simulink model "SingleVehicle_01"  (Simulink 8.8)
settings: Solver=ode45  StartTime=0.0  StopTime=17  RelTol=1e-3  EnableMultiTasking=on
undefined symbols (not defined in the file or in its folder): DiscIntNeverNeededParam, dpsi, FromPrescan, IdealSensors, psi, RHSC, RHSCCmdBus, unscented_KF_dd, v, wpFollower, y
undefined symbols (not defined in the file): vd
libraries: commchan3 x4
settings Model: Creator=sgopalswamy  LastModifiedBy=yutongli
settings SolverCC: AutoInsertRateTranBlk=on
settings DataIOCC: LimitDataPoints=off  SaveFormat=Dataset  SignalLoggingSaveFormat=Dataset
settings OptimizationCC: LifeSpan=auto
settings DebuggingCC: MultiTaskRateTransMsg=warning  FcnCallInpInsideContextMsg=error  StateNameClashWarn=none  SFUnexpectedBacktrackingDiag=error  SFNoUnconditionalDefaultTransitionDiag=error
settings HardwareCC: ProdBitPerPointer=64  ProdBitPerSizeT=64  ProdBitPerPtrDiffT=64  ProdLargestAtomicFloat=Float  ProdIntDivRoundTo=Zero  ProdEndianess=LittleEndian  ProdWordSize=64  ProdHWDeviceType=Intel->x86-64 (Windows64)
settings ModelReferenceCC: PropagateSignalLabelsOutOfModel=on
settings GRTTargetCC: TargetLangStandard=C99 (ISO)  GeneratePreprocessorConditionals=Use local settings  CombineOutputUpdateFcns=on  GRTInterface=off
settings ConfigComp: CovSFcnEnable=off

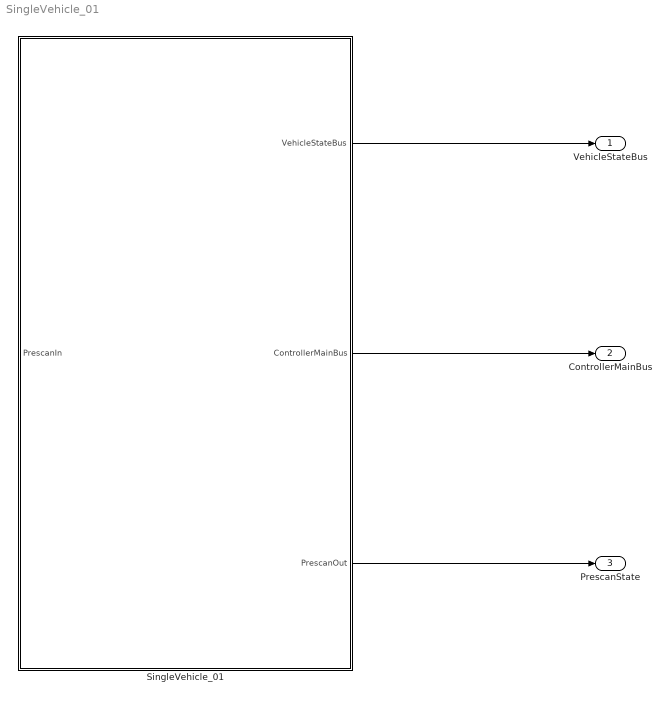
== system SingleVehicle_01 ==
  SingleVehicle_01 : Subsystem  mask{veh_struct=vd}
      mask prompts: veh_struct "Vehicle Parameter Structure"
      mask init:
      | set_param([gcb,'/Monitor/VehicleStateBusStorage'],'VariableName',[get_param(gcb,'MaskValueString'),'_DataVehicleBus']);
      | set_param([gcb,'/Monitor/ControllerMainBusStorage/ArbitratedActuationReqStorage'],'VariableName', ...
      |     [get_param(gcb,'MaskValueString'),'_DataControllerMain_ArbitrationActuationReq']);
      | set_param([gcb,'/Monitor/ControllerMainBusStorage/wpFollowerStorage'],'VariableName', ...
      |     [get_param(gcb,'MaskValueString'),'_DataControllerMain_wpFollower']);
      | set_param([gcb,'/Monitor/ControllerMainBusStorage/finalWayPointStorarge'],'VariableName', ...
      |     [get_param(gcb,'MaskValueString'),'_DataControllerMain_finalWayPoint']);
      | set_param([gcb,'/Monitor/ControllerMainBusStorage/currentWayPointStorage'],'VariableName', ...
      |     [get_param(gcb,'MaskValueString'),'_DataControllerMain_currentWayPoint']);
      | set_param([gcb,'/Monitor/ControllerMainBusStorage/wayPointArrayStorage'],'VariableName', ...
      |     [get_param(gcb,'MaskValueString'),'_DataControllerMain_wayPointArray']);
      | set_param([gcb,'/Monitor/ControllerMainBusStorage/selfAwareessBusStorage'],'VariableName', ...
      |     [get_param(gcb,'MaskValueString'),'_DataControllerMain_selfAwareessBus']);
      | set_param([gcb,'/Monitor/ControllerMainBusStorage/IdealSensorsStorage'],'VariableName', ...
      |     [get_param(gcb,'MaskValueString'),'_DataControllerMain_IdealSensors']);
      | set_param([gcb,'/Monitor/ControllerMainBusStorage/FromPrescanStorage'],'VariableName', ...
      |     [get_param(gcb,'MaskValueString'),'_DataControllerMain_FromPrescan']);
  VehicleStateBus : Outport
  ControllerMainBus : Outport  Port=2
  PrescanState : Outport  Port=3
  wires:
  SingleVehicle_01/1(VehicleStateBus) -> VehicleStateBus/1
  SingleVehicle_01/2(ControllerMainBus) -> ControllerMainBus/1
  SingleVehicle_01/3(PrescanOut) -> PrescanState/1

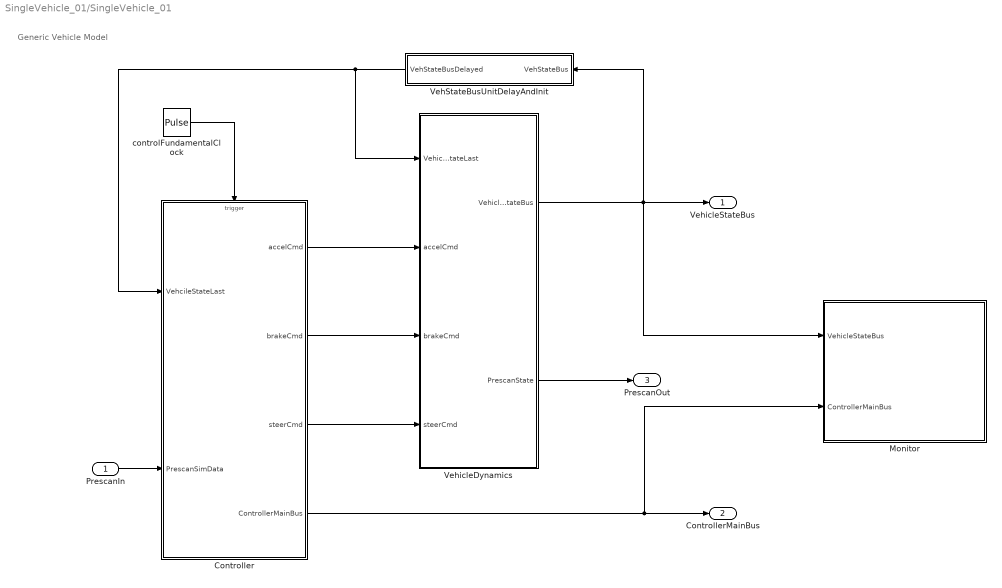
== system SingleVehicle_01/SingleVehicle_01 ==
  note: Generic Vehicle Model
  PrescanIn : Inport
  Controller : Subsystem
  Monitor : Subsystem
  VehStateBusUnitDelayAndInit : Subsystem
  VehicleDynamics : Subsystem
  controlFundamentalClock : DiscretePulseGenerator  PulseType=Time based  Period=veh_struct.CONTROL_OS_SAMPLETIME  PulseWidth=5
  VehicleStateBus : Outport
  ControllerMainBus : Outport  Port=2
  PrescanOut : Outport  Port=3
  wires:
  PrescanIn/1 -> Controller/2(PrescanSimData)
  Controller/1(accelCmd) -> VehicleDynamics/2(accelCmd)
  Controller/2(brakeCmd) -> VehicleDynamics/3(brakeCmd)
  Controller/3(steerCmd) -> VehicleDynamics/4(steerCmd)
  Controller/4(ControllerMainBus) -> Monitor/2(ControllerMainBus), ControllerMainBus/1
  VehicleDynamics/2(PrescanState) -> PrescanOut/1
  VehicleDynamics/1(VehicleStateBus) -> Monitor/1(VehicleStateBus), VehicleStateBus/1, VehStateBusUnitDelayAndInit/1(VehStateBus)
  VehStateBusUnitDelayAndInit/1(VehStateBusDelayed) -> VehicleDynamics/1(VehicleStateLast), Controller/1(VehcileStateLast)
  controlFundamentalClock/1 -> Controller/Trigger

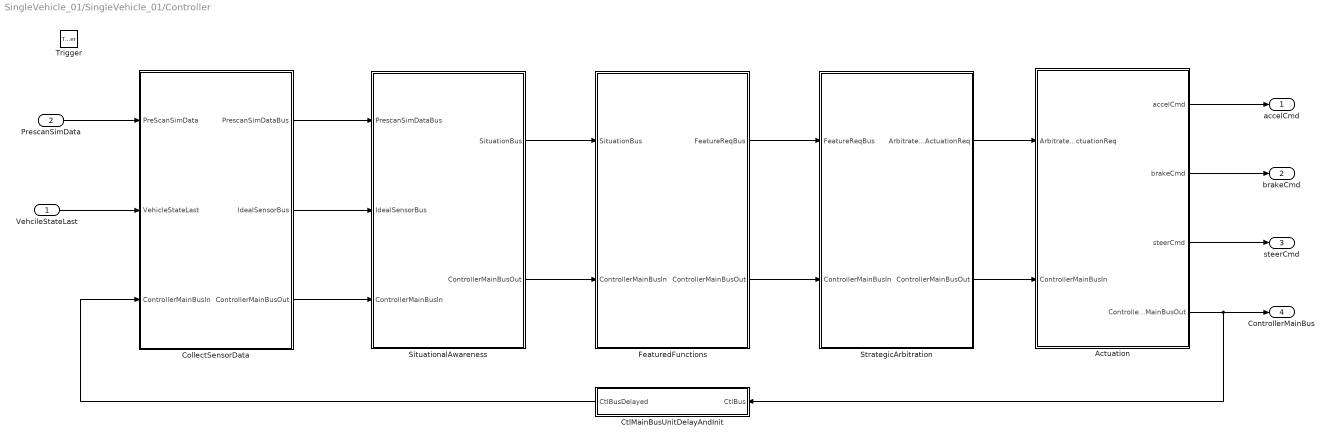
== system SingleVehicle_01/SingleVehicle_01/Controller ==
  VehcileStateLast : Inport
  PrescanSimData : Inport  Port=2
  Trigger : TriggerPort  VariantControl=Variant  PortDimensions=1
  Actuation : Subsystem
  CollectSensorData : Subsystem
  CtlMainBusUnitDelayAndInit : Subsystem
  FeaturedFunctions : Subsystem
  SituationalAwareness : Subsystem
  StrategicArbitration : Subsystem
  accelCmd : Outport
  brakeCmd : Outport  Port=2
  steerCmd : Outport  Port=3
  ControllerMainBus : Outport  Port=4
  wires:
  PrescanSimData/1 -> CollectSensorData/1(PreScanSimData)
  Actuation/1(accelCmd) -> accelCmd/1
  Actuation/2(brakeCmd) -> brakeCmd/1
  Actuation/3(steerCmd) -> steerCmd/1
  StrategicArbitration/1(ArbitratedActuationReq) -> Actuation/1(ArbitratedActuationReq)
  StrategicArbitration/2(ControllerMainBusOut) -> Actuation/2(ControllerMainBusIn)
  FeaturedFunctions/2(ControllerMainBusOut) -> StrategicArbitration/2(ControllerMainBusIn)
  FeaturedFunctions/1(FeatureReqBus) -> StrategicArbitration/1(FeatureReqBus)
  SituationalAwareness/1(SituationBus) -> FeaturedFunctions/1(SituationBus)
  SituationalAwareness/2(ControllerMainBusOut) -> FeaturedFunctions/2(ControllerMainBusIn)
  CollectSensorData/3(ControllerMainBusOut) -> SituationalAwareness/3(ControllerMainBusIn)
  VehcileStateLast/1 -> CollectSensorData/2(VehicleStateLast)
  Actuation/4(ControllerMainBusOut) -> CtlMainBusUnitDelayAndInit/1(CtlBus), ControllerMainBus/1
  CtlMainBusUnitDelayAndInit/1(CtlBusDelayed) -> CollectSensorData/3(ControllerMainBusIn)
  CollectSensorData/1(PrescanSimDataBus) -> SituationalAwareness/1(PrescanSimDataBus)
  CollectSensorData/2(IdealSensorBus) -> SituationalAwareness/2(IdealSensorBus)

== system SingleVehicle_01/SingleVehicle_01/Monitor ==
  VehicleStateBus : Inport
  ControllerMainBus : Inport  Port=2
  ControllerMainBusStorage : Subsystem
  VehicleStateBusStorage : ToWorkspace  VariableName=vd_DataVehicleBus  SaveFormat=Timeseries  SampleTime=-1
  wires:
  VehicleStateBus/1 -> VehicleStateBusStorage/1
  ControllerMainBus/1 -> ControllerMainBusStorage/1(ControllerMainBus)

== system SingleVehicle_01/SingleVehicle_01/VehStateBusUnitDelayAndInit ==
  VehStateBus : Inport
  MATLAB Function : MATLAB Function  TreatAsAtomicUnit=on
  Memory : Memory  InheritSampleTime=on
  VehStateBusDelayed : Outport
  wires:
  Memory/1 -> MATLAB Function/1(u)
  VehStateBus/1 -> Memory/1
  MATLAB Function/1(y) -> VehStateBusDelayed/1

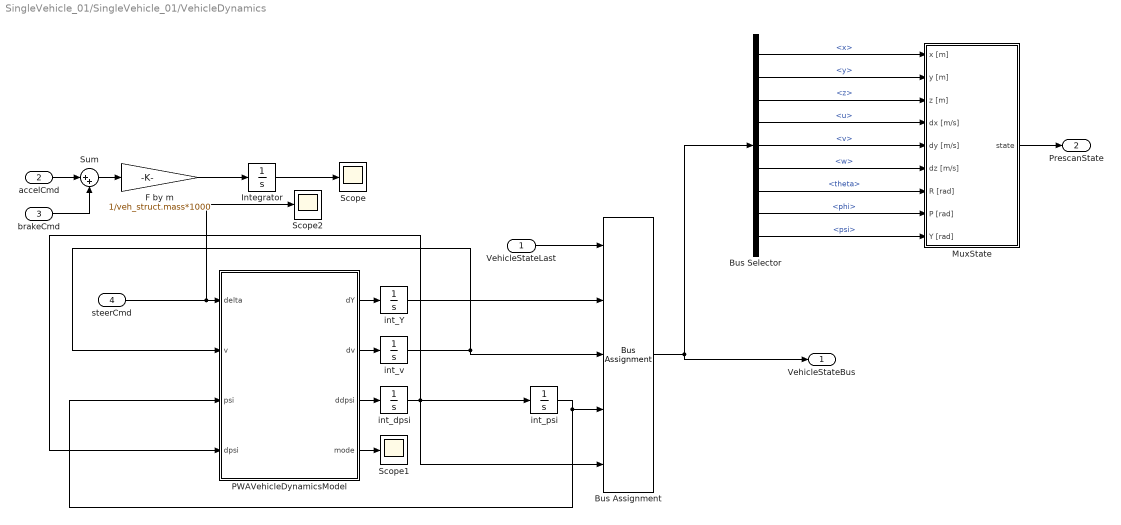
== system SingleVehicle_01/SingleVehicle_01/VehicleDynamics ==
  VehicleStateLast : Inport
  accelCmd : Inport  Port=2
  brakeCmd : Inport  Port=3
  steerCmd : Inport  Port=4
  Bus Assignment : BusAssignment  AssignedSignals=y,v,psi,dpsi
  Bus Selector : BusSelector  OutputSignals=x,y,z,u,v,w,theta,phi,psi
  F by m : Gain  Gain=1/veh_struct.mass*1000
  Integrator : Integrator  InitialCondition=veh_struct.init.u
  MuxState : Subsystem  Tag=MuxState  mask(Empty Dynamics State Block){positioningmode=on, TimeStep=1/20}
      mask prompts: positioningmode "Positioning Mode"; TimeStep "Auto Assigned: Time Step [s]"
      mask help:
      | Build the state of an actor based on user input.
      | The user can either use positioning mode or dynamics mode.
      | - When using positioning mode the position and orientation of the actor are set directly based on the input. Expected input is relative to the initial position and orientation of the actor. It's also possible to specify the velocity of the actor, though this input isn't used, only passed on.
      | - When using dynamics mode the position input is ignored. Expected input is velocity and orientation. The velocity is relative the current orientation of the actor, while orientation is relative to its initial orientation. The position of the actor is calculated based on the velocity and orientation given.
      settings: DeleteFcn=PreScanBlockDeleteFcn;
  PWAVehicleDynamicsModel : MATLAB Function  TreatAsAtomicUnit=on
  Scope : Scope
  Scope1 : Scope
  Scope2 : Scope
  Sum : Sum  Inputs=|++
  int_Y : Integrator  InitialCondition=veh_struct.init.Y
  int_dpsi : Integrator  InitialCondition=veh_struct.init.dpsi
  int_psi : Integrator  InitialCondition=veh_struct.init.psi
  int_v : Integrator  InitialCondition=veh_struct.init.v
  VehicleStateBus : Outport
  PrescanState : Outport  Port=2
  wires:
  MuxState/1(state) -> PrescanState/1
  Bus Assignment/1 -> VehicleStateBus/1, Bus Selector/1
  Bus Selector/3 -> MuxState/3(z [m])  "<z>"
  Bus Selector/4 -> MuxState/4(dx [m/s])  "<u>"
  Bus Selector/5 -> MuxState/5(dy [m/s])  "<v>"
  Bus Selector/6 -> MuxState/6(dz [m/s])  "<w>"
  Bus Selector/1 -> MuxState/1(x [m])  "<x>"
  Bus Selector/2 -> MuxState/2(y [m])  "<y>"
  Bus Selector/7 -> MuxState/7(R [rad])  "<theta>"
  Bus Selector/9 -> MuxState/9(Y [rad])  "<psi>"
  Bus Selector/8 -> MuxState/8(P [rad])  "<phi>"
  VehicleStateLast/1 -> Bus Assignment/1
  accelCmd/1 -> Sum/1
  brakeCmd/1 -> Sum/2
  Sum/1 -> F by m/1
  F by m/1 -> Integrator/1
  Integrator/1 -> Scope/1
  PWAVehicleDynamicsModel/2(dv) -> int_v/1
  int_v/1 -> Bus Assignment/3, PWAVehicleDynamicsModel/2(v)
  PWAVehicleDynamicsModel/3(ddpsi) -> int_dpsi/1
  int_dpsi/1 -> Bus Assignment/5, int_psi/1, PWAVehicleDynamicsModel/4(dpsi)
  PWAVehicleDynamicsModel/1(dY) -> int_Y/1
  int_Y/1 -> Bus Assignment/2
  int_psi/1 -> PWAVehicleDynamicsModel/3(psi), Bus Assignment/4
  PWAVehicleDynamicsModel/4(mode) -> Scope1/1
  steerCmd/1 -> Scope2/1, PWAVehicleDynamicsModel/1(delta)

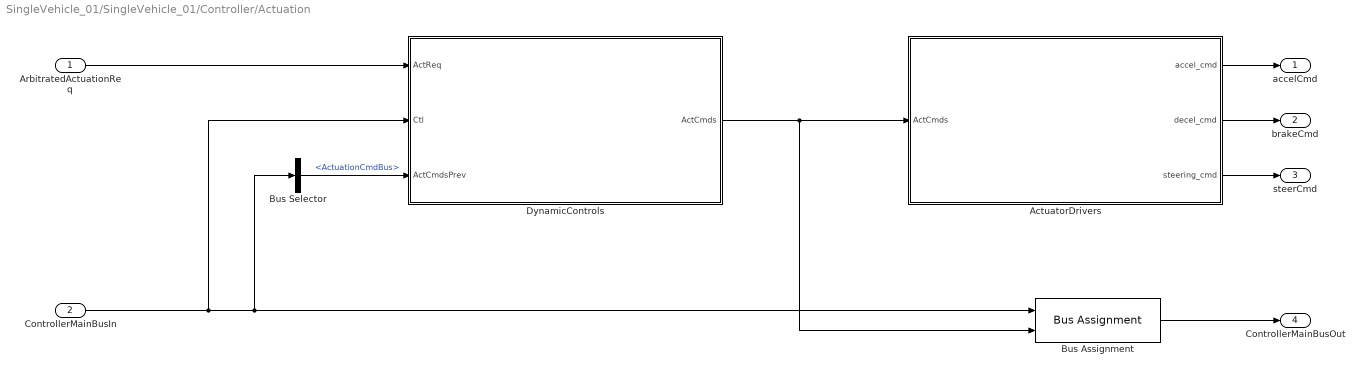
== system SingleVehicle_01/SingleVehicle_01/Controller/Actuation ==
  ArbitratedActuationReq : Inport
  ControllerMainBusIn : Inport  Port=2
  ActuatorDrivers : MATLAB Function  TreatAsAtomicUnit=on
  Bus Assignment : BusAssignment  AssignedSignals=ActuationCmdBus
  Bus Selector : BusSelector  OutputSignals=ActuationCmdBus
  DynamicControls : MATLAB Function  TreatAsAtomicUnit=on
  accelCmd : Outport
  brakeCmd : Outport  Port=2
  steerCmd : Outport  Port=3
  ControllerMainBusOut : Outport  Port=4
  wires:
  ControllerMainBusIn/1 -> DynamicControls/2(Ctl), Bus Assignment/1, Bus Selector/1
  ArbitratedActuationReq/1 -> DynamicControls/1(ActReq)
  Bus Selector/1 -> DynamicControls/3(ActCmdsPrev)  "<ActuationCmdBus>"
  DynamicControls/1(ActCmds) -> ActuatorDrivers/1(ActCmds), Bus Assignment/2
  Bus Assignment/1 -> ControllerMainBusOut/1
  ActuatorDrivers/2(decel_cmd) -> brakeCmd/1
  ActuatorDrivers/1(accel_cmd) -> accelCmd/1
  ActuatorDrivers/3(steering_cmd) -> steerCmd/1

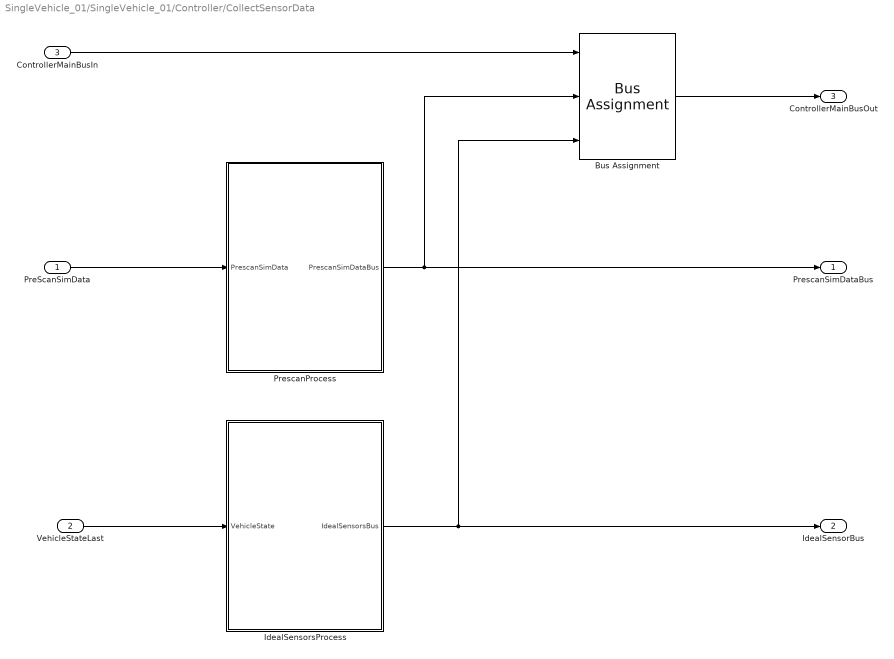
== system SingleVehicle_01/SingleVehicle_01/Controller/CollectSensorData ==
  PreScanSimData : Inport
  VehicleStateLast : Inport  Port=2
  ControllerMainBusIn : Inport  Port=3
  Bus Assignment : BusAssignment  AssignedSignals=FromPrescan,IdealSensors
  IdealSensorsProcess : Subsystem
  PrescanProcess : Subsystem
  PrescanSimDataBus : Outport
  IdealSensorBus : Outport  Port=2
  ControllerMainBusOut : Outport  Port=3
  wires:
  PreScanSimData/1 -> PrescanProcess/1(PrescanSimData)
  PrescanProcess/1(PrescanSimDataBus) -> Bus Assignment/2, PrescanSimDataBus/1
  VehicleStateLast/1 -> IdealSensorsProcess/1(VehicleState)
  IdealSensorsProcess/1(IdealSensorsBus) -> IdealSensorBus/1, Bus Assignment/3
  Bus Assignment/1 -> ControllerMainBusOut/1
  ControllerMainBusIn/1 -> Bus Assignment/1

== system SingleVehicle_01/SingleVehicle_01/Controller/CtlMainBusUnitDelayAndInit ==
  CtlBus : Inport
  MATLAB Function : MATLAB Function  TreatAsAtomicUnit=on
  Memory : Memory  InheritSampleTime=on
  CtlBusDelayed : Outport
  wires:
  Memory/1 -> MATLAB Function/1(u)
  CtlBus/1 -> Memory/1
  MATLAB Function/1(y) -> CtlBusDelayed/1

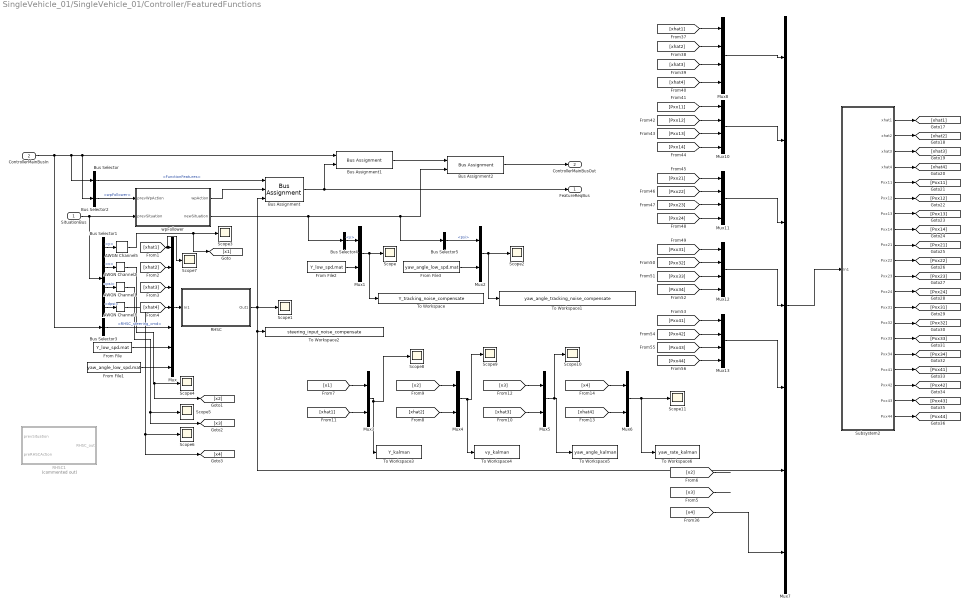
== system SingleVehicle_01/SingleVehicle_01/Controller/FeaturedFunctions ==
  SituationBus : Inport
  ControllerMainBusIn : Inport  Port=2
  AWGN Channel{1..3,5} (4 alike) : commchan3/AWGN Channel  InputProcessing=Columns as channels (frame based)  seed=67  noiseMode="Signal to noise ratio  (SNR)"  EbNodB=10  EsNodB=10  SNRdB=40  bitsPerSym=1  Ps=1  Tsym=1  variance=1
  Bus Assignment : BusAssignment  AssignedSignals=wpFollower,RHSCCmdBus.RHSC_steering_cmd
  Bus Assignment1 : BusAssignment  AssignedSignals=FunctionFeatures
  Bus Assignment2 : BusAssignment  AssignedSignals=situationBus
  Bus Selector : BusSelector  OutputSignals=FunctionFeatures
  Bus Selector1 : BusSelector  OutputSignals=selfAwarenessBus.y,selfAwarenessBus.v,selfAwarenessBus.psi,selfAwarenessBus.dpsi
  Bus Selector2 : BusSelector  OutputSignals=FunctionFeatures.wpFollower
  Bus Selector3 : BusSelector  OutputSignals=FunctionFeatures.RHSCCmdBus.RHSC_steering_cmd
  Bus Selector4 : BusSelector  OutputSignals=selfAwarenessBus.y
  Bus Selector5 : BusSelector  OutputSignals=selfAwarenessBus.psi
  From File : FromFile  FileName=Y_low_spd.mat
  From File1 : FromFile  FileName=yaw_angle_low_spd.mat
  From File2 : FromFile  FileName=Y_low_spd.mat
  From File3 : FromFile  FileName=yaw_angle_low_spd.mat
  Mux : Mux  Inputs=7
  Mux{1..6} (6 alike) : Mux  Inputs=2
  Mux{8,10..13} (5 alike) : Mux
  Mux7 : Mux  Inputs=7
  RHSC : Subsystem
  RHSC1 : MATLAB Function  Commented=on  TreatAsAtomicUnit=on
  Scope{,1..11} (12 alike) : Scope
  Subsystem2 : Subsystem
  To Workspace : ToWorkspace  VariableName=Y_tracking_noise_compensate  SaveFormat=Timeseries  SampleTime=-1
  To Workspace1 : ToWorkspace  VariableName=yaw_angle_tracking_noise_compensate  SaveFormat=Timeseries  SampleTime=-1
  To Workspace2 : ToWorkspace  VariableName=steering_input_noise_compensate  SaveFormat=Timeseries  SampleTime=-1
  To Workspace3 : ToWorkspace  VariableName=Y_kalman  SaveFormat=Timeseries  SampleTime=-1
  To Workspace4 : ToWorkspace  VariableName=vy_kalman  SaveFormat=Timeseries  SampleTime=-1
  To Workspace5 : ToWorkspace  VariableName=yaw_angle_kalman  SaveFormat=Timeseries  SampleTime=-1
  To Workspace6 : ToWorkspace  VariableName=yaw_rate_kalman  SaveFormat=Timeseries  SampleTime=-1
  wpFollower : MATLAB Function  TreatAsAtomicUnit=on
  FeatureReqBus : Outport
  ControllerMainBusOut : Outport  Port=2
  wires:
  ControllerMainBusIn/1 -> Bus Selector3/1, Bus Selector/1, Bus Selector2/1, Bus Assignment1/1
  Bus Selector/1 -> Bus Assignment/1  "<FunctionFeatures>"
  wpFollower/1(wpAction) -> Bus Assignment/2
  Bus Assignment/1 -> Bus Assignment1/2, FeatureReqBus/1
  Bus Assignment1/1 -> Bus Assignment2/1
  wpFollower/2(newSituation) -> Bus Selector4/1, Bus Selector5/1, Bus Assignment2/2
  Bus Assignment2/1 -> ControllerMainBusOut/1
  Bus Selector2/1 -> wpFollower/1(prevWpAction)  "<wpFollower>"
  SituationBus/1 -> Bus Selector1/1, wpFollower/2(prevSituation)
  Bus Selector3/1 -> Mux/5  "<RHSC_steering_cmd>"
  Mux/1 -> RHSC/1(In1)
  Bus Selector1/1 -> AWGN Channel5/1  "<y>"
  Bus Selector1/2 -> AWGN Channel2/1  "<v>"
  Bus Selector1/3 -> AWGN Channel1/1  "<psi>"
  Bus Selector1/4 -> AWGN Channel3/1  "<dpsi>"
  From File/1 -> Mux/6
  From File1/1 -> Mux/7
  Bus Selector4/1 -> Mux1/1  "<y>"
  From File2/1 -> Mux1/2
  Mux1/1 -> To Workspace/1, Scope/1
  Bus Selector5/1 -> Mux2/1  "<psi>"
  From File3/1 -> Mux2/2
  Mux2/1 -> To Workspace1/1, Scope2/1
  Mux7/1 -> Subsystem2/1(In1)
  Mux8/1 -> Mux7/1
  Mux10/1 -> Mux7/2
  Mux11/1 -> Mux7/3
  Mux12/1 -> Mux7/4
  Mux13/1 -> Mux7/5
  Subsystem2/1(xhat1) -> [xhat1]
  Subsystem2/2(xhat2) -> [xhat2]
  Subsystem2/3(xhat3) -> [xhat3]
  Subsystem2/4(xhat4) -> [xhat4]
  Subsystem2/5(Pxx11) -> [Pxx11]
  Subsystem2/6(Pxx12) -> [Pxx12]
  Subsystem2/7(Pxx13) -> [Pxx13]
  Subsystem2/8(Pxx14) -> [Pxx14]
  Subsystem2/9(Pxx21) -> [Pxx21]
  Subsystem2/10(Pxx22) -> [Pxx22]
  Subsystem2/11(Pxx23) -> [Pxx23]
  Subsystem2/12(Pxx24) -> [Pxx24]
  Subsystem2/13(Pxx31) -> [Pxx31]
  Subsystem2/14(Pxx32) -> [Pxx32]
  Subsystem2/15(Pxx33) -> [Pxx33]
  Subsystem2/16(Pxx34) -> [Pxx34]
  Subsystem2/17(Pxx41) -> [Pxx41]
  Subsystem2/18(Pxx42) -> [Pxx42]
  Subsystem2/19(Pxx43) -> [Pxx43]
  Subsystem2/20(Pxx44) -> [Pxx44]
  [xhat1] -> Mux8/1
  [xhat2] -> Mux8/2
  [xhat3] -> Mux8/3
  [xhat4] -> Mux8/4
  [Pxx11] -> Mux10/1
  [Pxx12] -> Mux10/2
  [Pxx13] -> Mux10/3
  [Pxx14] -> Mux10/4
  [Pxx21] -> Mux11/1
  [Pxx22] -> Mux11/2
  [Pxx23] -> Mux11/3
  [Pxx24] -> Mux11/4
  [Pxx31] -> Mux12/1
  [Pxx32] -> Mux12/2
  [Pxx33] -> Mux12/3
  [Pxx34] -> Mux12/4
  [Pxx41] -> Mux13/1
  [Pxx42] -> Mux13/2
  [Pxx43] -> Mux13/3
  [Pxx44] -> Mux13/4
  RHSC/1(Out1) -> Mux7/6, To Workspace2/1, Scope1/1, Bus Assignment/3
  [xhat1] -> Scope7/1, Mux/1
  [xhat2] -> Mux/2
  [xhat3] -> Mux/3
  [xhat4] -> Mux/4
  [x4] -> Mux7/7
  [x1] -> Mux3/1
  [x2] -> ?
  [x3] -> ?
  AWGN Channel5/1 -> [x1], Scope3/1
  AWGN Channel1/1 -> [x3], Scope5/1
  AWGN Channel2/1 -> [x2], Scope4/1
  AWGN Channel3/1 -> [x4], Scope6/1
  [xhat1] -> Mux3/2
  [x2] -> Mux4/1
  [xhat2] -> Mux4/2
  [x3] -> Mux5/1
  [xhat3] -> Mux5/2
  [x4] -> Mux6/1
  [xhat4] -> Mux6/2
  Mux3/1 -> Scope8/1, To Workspace3/1
  Mux4/1 -> Scope9/1, To Workspace4/1
  Mux5/1 -> Scope10/1, To Workspace5/1
  Mux6/1 -> Scope11/1, To Workspace6/1

== system SingleVehicle_01/SingleVehicle_01/Controller/SituationalAwareness ==
  PrescanSimDataBus : Inport
  IdealSensorBus : Inport  Port=2
  ControllerMainBusIn : Inport  Port=3
  Bus Assignment : BusAssignment  AssignedSignals=situationBus
  Bus Selector : BusSelector  OutputSignals=situationBus
  situationAwareness : MATLAB Function  TreatAsAtomicUnit=on
  SituationBus : Outport
  ControllerMainBusOut : Outport  Port=2
  wires:
  ControllerMainBusIn/1 -> Bus Assignment/1, Bus Selector/1
  Bus Selector/1 -> situationAwareness/1(prevSituation)  "<situationBus>"
  PrescanSimDataBus/1 -> situationAwareness/2(prescanSimData)
  IdealSensorBus/1 -> situationAwareness/3(idealSensors)
  situationAwareness/1(newSituation) -> Bus Assignment/2, SituationBus/1
  Bus Assignment/1 -> ControllerMainBusOut/1

== system SingleVehicle_01/SingleVehicle_01/Controller/StrategicArbitration ==
  FeatureReqBus : Inport
  ControllerMainBusIn : Inport  Port=2
  Arbitration : MATLAB Function  TreatAsAtomicUnit=on
  Bus Assignment : BusAssignment  AssignedSignals=ArbitratedActuationReq
  ArbitratedActuationReq : Outport
  ControllerMainBusOut : Outport  Port=2
  wires:
  FeatureReqBus/1 -> Arbitration/1(FunctionFeatures)
  Arbitration/1(ArbitratedReq) -> Bus Assignment/2, ArbitratedActuationReq/1
  ControllerMainBusIn/1 -> Bus Assignment/1
  Bus Assignment/1 -> ControllerMainBusOut/1

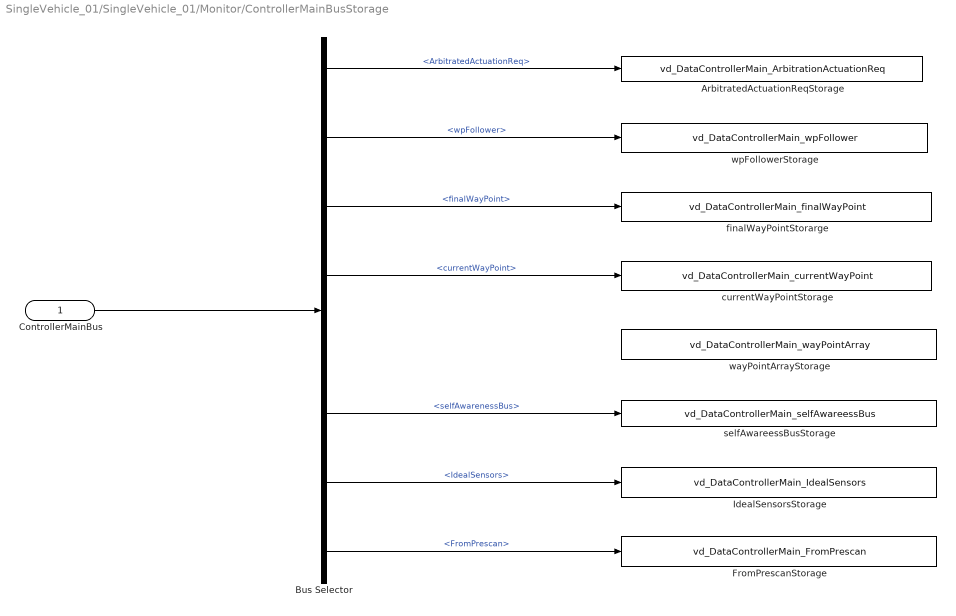
== system SingleVehicle_01/SingleVehicle_01/Monitor/ControllerMainBusStorage ==
  ControllerMainBus : Inport
  ArbitratedActuationReqStorage : ToWorkspace  VariableName=vd_DataControllerMain_ArbitrationActuationReq  SaveFormat=Timeseries  SampleTime=-1
  Bus Selector : BusSelector  OutputSignals=ArbitratedActuationReq,FunctionFeatures.wpFollower,situationBus.wP.finalWayPoint,situationBus.wP.currentWayPoint,situationBus.wP.wayPointArray,situationBus.selfAwarenessBus,IdealSensors,FromPrescan
  FromPrescanStorage : ToWorkspace  VariableName=vd_DataControllerMain_FromPrescan  SaveFormat=Timeseries  SampleTime=-1
  IdealSensorsStorage : ToWorkspace  VariableName=vd_DataControllerMain_IdealSensors  SaveFormat=Timeseries  SampleTime=-1
  currentWayPointStorage : ToWorkspace  VariableName=vd_DataControllerMain_currentWayPoint  SaveFormat=Timeseries  SampleTime=-1
  finalWayPointStorarge : ToWorkspace  VariableName=vd_DataControllerMain_finalWayPoint  SaveFormat=Timeseries  SampleTime=-1
  selfAwareessBusStorage : ToWorkspace  VariableName=vd_DataControllerMain_selfAwareessBus  SaveFormat=Timeseries  SampleTime=-1
  wayPointArrayStorage : ToWorkspace  VariableName=vd_DataControllerMain_wayPointArray  SampleTime=-1
  wpFollowerStorage : ToWorkspace  VariableName=vd_DataControllerMain_wpFollower  SaveFormat=Timeseries  SampleTime=-1
  wires:
  ControllerMainBus/1 -> Bus Selector/1
  Bus Selector/1 -> ArbitratedActuationReqStorage/1  "<ArbitratedActuationReq>"
  Bus Selector/2 -> wpFollowerStorage/1  "<wpFollower>"
  Bus Selector/3 -> finalWayPointStorarge/1  "<finalWayPoint>"
  Bus Selector/8 -> FromPrescanStorage/1  "<FromPrescan>"
  Bus Selector/6 -> selfAwareessBusStorage/1  "<selfAwarenessBus>"
  Bus Selector/4 -> currentWayPointStorage/1  "<currentWayPoint>"
  Bus Selector/7 -> IdealSensorsStorage/1  "<IdealSensors>"

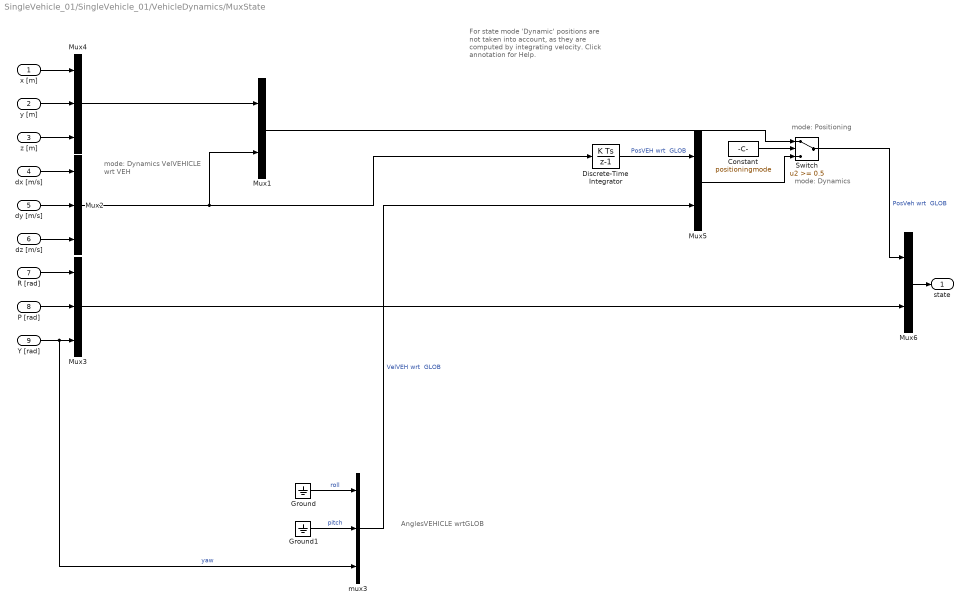
== system SingleVehicle_01/SingleVehicle_01/VehicleDynamics/MuxState ==
  note: mode: Dynamics
  note: mode: Positioning
  note: mode: Dynamics
      | VelVEHICLE
      | wrt VEH
  note: AnglesVEHICLE
      | wrtGLOB
  note: For state mode 'Dynamic' positions
      | are not taken into account, as they
      | are computed by integrating velocity.
      | Click annotation for Help.
  x [m] : Inport  SampleTime=TimeStep
  y [m] : Inport  Port=2  SampleTime=TimeStep
  z [m] : Inport  Port=3  SampleTime=TimeStep
  dx [m/s] : Inport  Port=4  SampleTime=TimeStep
  dy [m/s] : Inport  Port=5  SampleTime=TimeStep
  dz [m/s] : Inport  Port=6  SampleTime=TimeStep
  R [rad] : Inport  Port=7  SampleTime=TimeStep
  P [rad] : Inport  Port=8  SampleTime=TimeStep
  Y [rad] : Inport  Port=9  SampleTime=TimeStep
  Constant : Constant  DisableCoverage=on  Value=positioningmode
  Discrete-Time Integrator : DiscreteIntegrator  SampleTime=TimeStep  ICPrevOutput=DiscIntNeverNeededParam  ICPrevScaledInput=DiscIntNeverNeededParam
  Ground : Ground
  Ground1 : Ground
  Mux1 : Mux  Inputs=[3 3]
  Mux2 : Mux  Inputs=3
  Mux3 : Mux  Inputs=3
  Mux4 : Mux  Inputs=3
  Mux5 : Mux  Inputs=[3 3]
  Mux6 : Mux  Inputs=[6 3]
  Switch : Switch  Threshold=0.5
  mux3 : Mux  Inputs=3
  state : Outport
  wires:
  Constant/1 -> Switch/2
  Mux6/1 -> state/1
  Mux4/1 -> Mux1/1
  Mux5/1 -> Switch/3
  Mux1/1 -> Switch/1
  Switch/1 -> Mux6/1  "PosVeh wrt  GLOB"
  P [rad]/1 -> Mux3/2
  R [rad]/1 -> Mux3/1
  dz [m/s]/1 -> Mux2/3
  dy [m/s]/1 -> Mux2/2
  dx [m/s]/1 -> Mux2/1
  z [m]/1 -> Mux4/3
  y [m]/1 -> Mux4/2
  x [m]/1 -> Mux4/1
  Ground1/1 -> mux3/2  "pitch"
  Y [rad]/1 -> mux3/3, Mux3/3  "yaw"
  Mux3/1 -> Mux6/2
  mux3/1 -> Mux5/2  "VelVEH wrt  GLOB"
  Ground/1 -> mux3/1  "roll"
  Mux2/1 -> Discrete-Time Integrator/1, Mux1/2
  Discrete-Time Integrator/1 -> Mux5/1  "PosVEH wrt  GLOB"

== system SingleVehicle_01/SingleVehicle_01/Controller/CollectSensorData/IdealSensorsProcess ==
  VehicleState : Inport
  Bus Creator : BusCreator  Inputs=12  OutDataTypeStr=Bus: VehState
  Bus Selector : BusSelector  OutputSignals=x,y,z,theta,phi,psi,u,v,w,dtheta,dphi,dpsi
  IdealSensorsBus : Outport
  wires:
  VehicleState/1 -> Bus Selector/1
  Bus Selector/1 -> Bus Creator/1  "<x>"
  Bus Selector/8 -> Bus Creator/8  "<v>"
  Bus Selector/7 -> Bus Creator/7  "<u>"
  Bus Selector/10 -> Bus Creator/10  "<dtheta>"
  Bus Selector/11 -> Bus Creator/11  "<dphi>"
  Bus Selector/6 -> Bus Creator/6  "<psi>"
  Bus Selector/4 -> Bus Creator/4  "<theta>"
  Bus Selector/9 -> Bus Creator/9  "<w>"
  Bus Selector/2 -> Bus Creator/2  "<y>"
  Bus Selector/5 -> Bus Creator/5  "<phi>"
  Bus Selector/12 -> Bus Creator/12  "<dpsi>"
  Bus Selector/3 -> Bus Creator/3  "<z>"
  Bus Creator/1 -> IdealSensorsBus/1

== system SingleVehicle_01/SingleVehicle_01/Controller/CollectSensorData/PrescanProcess ==
  PrescanSimData : Inport
  Bus Creator : BusCreator  Inputs=12  OutDataTypeStr=Bus: PrescanSimData
  SELF_Demux : Subsystem  Tag=DemuxSELF  mask(PreScan Demux Block:){}
      settings: DeleteFcn=PreScanBlockDeleteFcn;
      mask Display:
      | port_label('output',1,'x [m]')
      | port_label('output',2,'y [m]')
      | port_label('output',3,'z [m]','texmode','on')
      | port_label('output',4,'Rotx [deg]','texmode','on')
      | port_label('output',5,'Roty [deg]','texmode','on')
      | port_label('output',6,'Rotz [deg]','texmode','on')
      | port_label('output',7,'GPS lat [deg]','texmode','on')
      | port_label('output',8,'GPS long [deg]','texmode','on')
      | port_label('output',9,'GPS alt [m]','texmode','on')
      | port_label('output',10,'Velocity [m/s]')
      | port_label('output',11,'Heading [deg]')
      | port_label('output',12,'Yaw rate [deg/s]')
  PrescanSimDataBus : Outport
  wires:
  SELF_Demux/1(x [m]) -> Bus Creator/1  "x"
  PrescanSimData/1 -> SELF_Demux/1(SELF)
  Bus Creator/1 -> PrescanSimDataBus/1
  SELF_Demux/2(y [m]) -> Bus Creator/2  "y"
  SELF_Demux/3(z [m]) -> Bus Creator/3  "z"
  SELF_Demux/4(rotx [deg]) -> Bus Creator/4  "Rotx"
  SELF_Demux/5(roty [deg]) -> Bus Creator/5  "Roty"
  SELF_Demux/9(GPS alt [m]) -> Bus Creator/9  "GPS_alt"
  SELF_Demux/8(GPS long [deg]) -> Bus Creator/8  "GPS_long"
  SELF_Demux/10(velocity [m/s]) -> Bus Creator/10  "u"
  SELF_Demux/6(rotz [deg]) -> Bus Creator/6  "Rotz"
  SELF_Demux/7(GPS lat [deg]) -> Bus Creator/7  "GPS_lat"
  SELF_Demux/11(heading [deg]) -> Bus Creator/11  "heading"
  SELF_Demux/12(yaw rate [deg/s]) -> Bus Creator/12  "Yaw_rate"

== system SingleVehicle_01/SingleVehicle_01/Controller/FeaturedFunctions/RHSC ==
  In1 : Inport  PortDimensions=7
  Interpreted MATLAB Function : MATLABFcn  MATLABFcn=RHSC(u(1),u(2),u(3),u(4),u(5),u(6),u(7))
  Out1 : Outport
  wires:
  In1/1 -> Interpreted MATLAB Function/1
  Interpreted MATLAB Function/1 -> Out1/1

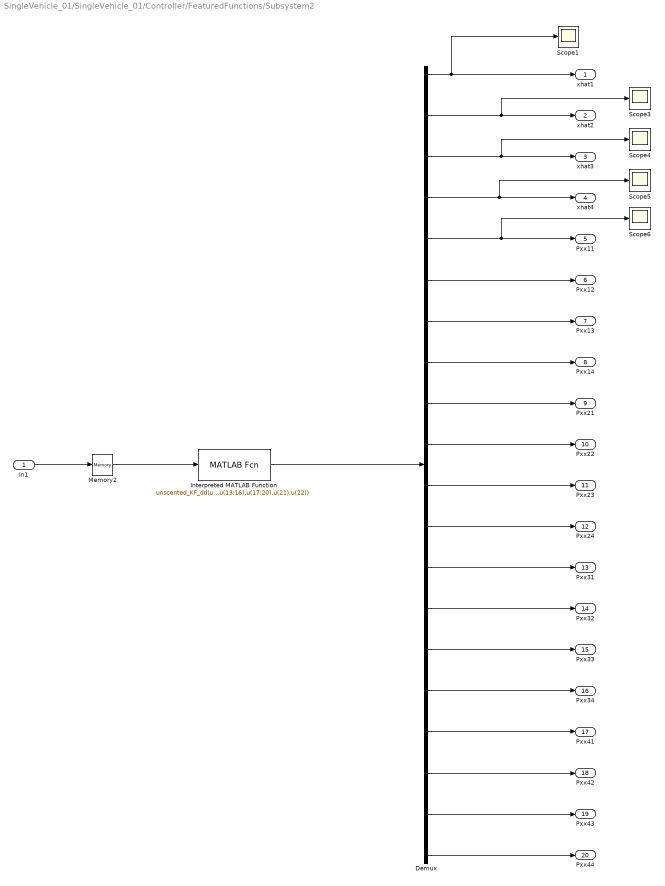
== system SingleVehicle_01/SingleVehicle_01/Controller/FeaturedFunctions/Subsystem2 ==
  In1 : Inport  PortDimensions=22
  Demux : Demux  Outputs=20
  Interpreted MATLAB Function : MATLABFcn  MATLABFcn=unscented_KF_dd(u(1:4),u(5:8),u(9:12),u(13:16),u(17:20),u(21),u(22))  OutputDimensions=20  Output1D=off
  Memory2 : Memory  InheritSampleTime=on
  Scope{1,3..6} (5 alike) : Scope
  xhat1 : Outport  PortDimensions=1
  xhat2 : Outport  Port=2  PortDimensions=1
  xhat3 : Outport  Port=3  PortDimensions=1
  xhat4 : Outport  Port=4  PortDimensions=1
  Pxx11 : Outport  Port=5  PortDimensions=1
  Pxx12 : Outport  Port=6  PortDimensions=1
  Pxx13 : Outport  Port=7  PortDimensions=1
  Pxx14 : Outport  Port=8  PortDimensions=1
  Pxx21 : Outport  Port=9  PortDimensions=1
  Pxx22 : Outport  Port=10  PortDimensions=1
  Pxx23 : Outport  Port=11  PortDimensions=1
  Pxx24 : Outport  Port=12  PortDimensions=1
  Pxx31 : Outport  Port=13  PortDimensions=1
  Pxx32 : Outport  Port=14  PortDimensions=1
  Pxx33 : Outport  Port=15  PortDimensions=1
  Pxx34 : Outport  Port=16  PortDimensions=1
  Pxx41 : Outport  Port=17  PortDimensions=1
  Pxx42 : Outport  Port=18  PortDimensions=1
  Pxx43 : Outport  Port=19  PortDimensions=1
  Pxx44 : Outport  Port=20  PortDimensions=1
  wires:
  Demux/2 -> Scope3/1, xhat2/1
  Demux/1 -> Scope1/1, xhat1/1
  Demux/3 -> xhat3/1, Scope4/1
  Demux/4 -> xhat4/1, Scope5/1
  Demux/5 -> Pxx11/1, Scope6/1
  Demux/6 -> Pxx12/1
  Demux/7 -> Pxx13/1
  Demux/8 -> Pxx14/1
  Demux/9 -> Pxx21/1
  Demux/10 -> Pxx22/1
  Demux/11 -> Pxx23/1
  Demux/12 -> Pxx24/1
  Demux/13 -> Pxx31/1
  Demux/14 -> Pxx32/1
  Demux/15 -> Pxx33/1
  Demux/16 -> Pxx34/1
  Demux/17 -> Pxx41/1
  Demux/18 -> Pxx42/1
  Demux/19 -> Pxx43/1
  Demux/20 -> Pxx44/1
  In1/1 -> Memory2/1
  Interpreted MATLAB Function/1 -> Demux/1
  Memory2/1 -> Interpreted MATLAB Function/1

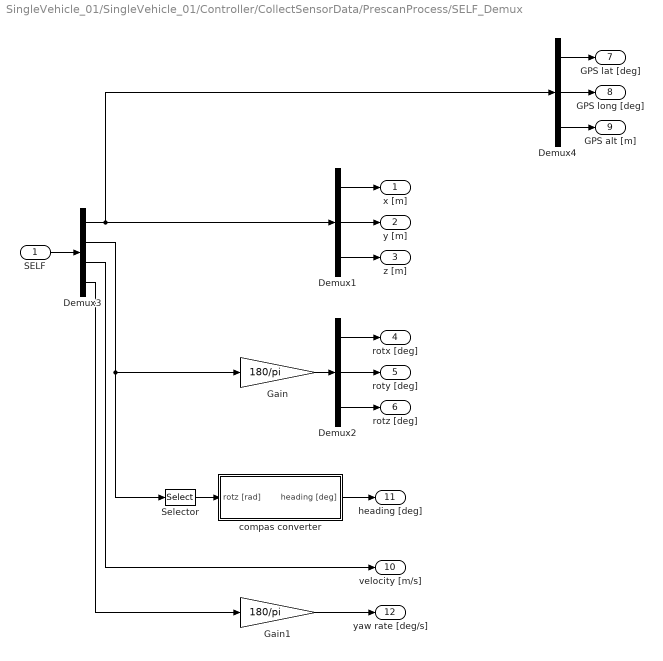
== system SingleVehicle_01/SingleVehicle_01/Controller/CollectSensorData/PrescanProcess/SELF_Demux ==
  SELF : Inport
  Demux1 : Demux  Outputs=3
  Demux2 : Demux  Outputs=3
  Demux3 : Demux  Outputs=[3 3 1 1]
  Demux4 : Demux  Outputs=3
  Gain : Gain  Gain=180/pi
  Gain1 : Gain  Gain=180/pi
  Selector : Selector  InputPortWidth=3  IndexOptions=Index vector (dialog)  Indices=[3]  OutputSizes=1
  compas converter : Subsystem
  x [m] : Outport
  y [m] : Outport  Port=2
  z [m] : Outport  Port=3
  rotx [deg] : Outport  Port=4
  roty [deg] : Outport  Port=5
  rotz [deg] : Outport  Port=6
  GPS lat [deg] : Outport  Port=7
  GPS long [deg] : Outport  Port=8
  GPS alt [m] : Outport  Port=9
  velocity [m/s] : Outport  Port=10
  heading [deg] : Outport  Port=11
  yaw rate [deg/s] : Outport  Port=12
  wires:
  Demux3/4 -> Gain1/1
  Gain1/1 -> yaw rate [deg/s]/1
  Demux3/3 -> velocity [m/s]/1
  compas converter/1(heading [deg]) -> heading [deg]/1
  Demux3/1 -> Demux4/1, Demux1/1
  Demux4/3 -> GPS alt [m]/1
  Demux4/2 -> GPS long [deg]/1
  Demux4/1 -> GPS lat [deg]/1
  Demux3/2 -> Gain/1, Selector/1
  SELF/1 -> Demux3/1
  Demux2/3 -> rotz [deg]/1
  Demux2/2 -> roty [deg]/1
  Demux2/1 -> rotx [deg]/1
  Demux1/3 -> z [m]/1
  Demux1/2 -> y [m]/1
  Demux1/1 -> x [m]/1
  Gain/1 -> Demux2/1
  Selector/1 -> compas converter/1(rotz [rad])

== system SingleVehicle_01/SingleVehicle_01/Controller/CollectSensorData/PrescanProcess/SELF_Demux/compas converter ==
  rotz [rad] : Inport
  cart2compas : Subsystem
  rad2deg : Gain  Gain=180/pi
  heading [deg] : Outport
  wires:
  cart2compas/1(heading [deg]) -> heading [deg]/1
  rotz [rad]/1 -> rad2deg/1
  rad2deg/1 -> cart2compas/1(Angle [deg])

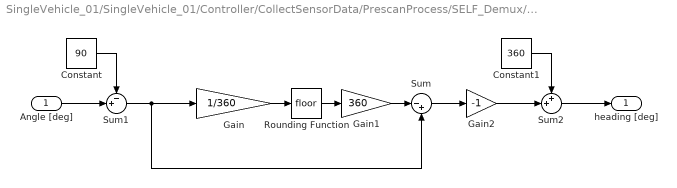
== system SingleVehicle_01/SingleVehicle_01/Controller/CollectSensorData/PrescanProcess/SELF_Demux/compas converter/cart2compas ==
  Angle [deg] : Inport
  Constant : Constant  Value=90
  Constant1 : Constant  Value=360
  Gain : Gain  Gain=1/360
  Gain1 : Gain  Gain=360
  Gain2 : Gain  Gain=-1
  Rounding Function : Rounding
  Sum : Sum  Inputs=|-+
  Sum1 : Sum  Inputs=-+|
  Sum2 : Sum  Inputs=++|
  heading [deg] : Outport
  wires:
  Sum2/1 -> heading [deg]/1
  Constant1/1 -> Sum2/1
  Gain2/1 -> Sum2/2
  Constant/1 -> Sum1/1
  Sum1/1 -> Sum/2, Gain/1
  Sum/1 -> Gain2/1
  Angle [deg]/1 -> Sum1/2
  Gain1/1 -> Sum/1
  Rounding Function/1 -> Gain1/1
  Gain/1 -> Rounding Function/1

== matlab function SingleVehicle_01/Controller/CtlMainBusUnitDelayAndInit/MATLAB Function ==
  data: u input double; y output Bus: ControllerMainBus; veh_struct parameter double
function y = DelayAndInitCtlBus(u, veh_struct)
coder.extrinsic('exist')
persistent a

y0 = struct;

y0.ActuationCmdBus = struct;
y0.ActuationCmdBus.steering_cmd = 0;
y0.ActuationCmdBus.decel_cmd = 0;
y0.ActuationCmdBus.accel_cmd = 0;



y0.ArbitratedActuationReq = struct;
y0.ArbitratedActuationReq.RHSCCmdBus = struct;
y0.ArbitratedActuationReq.RHSCCmdBus.RHSC_steering_cmd = 0;
y0.ArbitratedActuationReq.v_des = 0;
y0.ArbitratedActuationReq.a_des = 0;
y0.ArbitratedActuationReq.psi_des = 0;
y0.ArbitratedActuationReq.dpsi_des = 0;



y0.FunctionFeatures = struct;
y0.FunctionFeatures.RHSCCmdBus = struct;
y0.FunctionFeatures.RHSCCmdBus.RHSC_steering_cmd = 0;
y0.FunctionFeatures.wpFollower = struct;
y0.FunctionFeatures.wpFollower.v_des = 0;
y0.FunctionFeatures.wpFollower.a_des = 0;
y0.FunctionFeatures.wpFollower.psi_des = 0;
y0.FunctionFeatures.wpFollower.dpsi_des = 0;



y0.situationBus = struct;
y0.situationBus.wP = struct;

y0.situationBus.wP.finalWayPoint = struct;
y0.situationBus.wP.finalWayPoint.x = 0;
y0.situationBus.wP.finalWayPoint.y = 0;
y0.situationBus.wP.finalWayPoint.z = 0;
y0.situationBus.wP.finalWayPoint.treach = 0;

y0.situationBus.wP.currentWayPoint = struct;
y0.situationBus.wP.currentWayPoint.x = 0;
y0.situationBus.wP.currentWayPoint.y = 0;
y0.situationBus.wP.currentWayPoint.z = 0;
y0.situationBus.wP.currentWayPoint.treach = 0;

y0.situationBus.wP.finalWayPointIndex = uint16(1);
y0.situationBus.wP.currentWayPointIndex = uint16(10);

%y0.situationBus.wP.wayPointArray = struct;
wPArray = struct;
wPArray.x = 0;
wPArray.y = 0;
wPArray.z = 0;
wPArray.treach = 0;
y0.situationBus.wP.wayPointArray = repmat(wPArray,100,1);


y0.situationBus.selfAwarenessBus = struct;
y0.situationBus.selfAwarenessBus.x = 0;
y0.situationBus.selfAwarenessBus.y = 0;
y0.situationBus.selfAwarenessBus.z = 0;
y0.situationBus.selfAwarenessBus.theta = 0;
y0.situationBus.selfAwarenessBus.phi = 0;
y0.situationBus.selfAwarenessBus.psi = 0;
y0.situationBus.selfAwarenessBus.u = 0;
y0.situationBus.selfAwarenessBus.v = 0;
y0.situationBus.selfAwarenessBus.w = 0;
y0.situationBus.selfAwarenessBus.dtheta = 0;
y0.situationBus.selfAwarenessBus.dphi = 0;
y0.situationBus.selfAwarenessBus.dpsi = 0;
y0.IdealSensors = struct;
y0.IdealSensors.x = 0;
y0.IdealSensors.y = 0;
y0.IdealSensors.z = 0;
y0.IdealSensors.theta = 0;
y0.IdealSensors.phi = 0;
y0.IdealSensors.psi = 0;
y0.IdealSensors.u = 0;
y0.IdealSensors.v = 0;
y0.IdealSensors.w = 0;
y0.IdealSensors.dtheta = 0;
y0.IdealSensors.dphi = 0;
y0.IdealSensors.dpsi = 0;
y0.FromPrescan = struct;
y0.FromPrescan.x = 0;
y0.FromPrescan.y = 0;
y0.FromPrescan.z = 0;
y0.FromPrescan.Rotx = 0;
y0.FromPrescan.Roty = 0;
y0.FromPrescan.Rotz = 0;
y0.FromPrescan.GPS_lat = 0;
y0.FromPrescan.GPS_long = 0;
y0.FromPrescan.u = 0;
y0.FromPrescan.GPS_alt = 0;
y0.FromPrescan.heading = 0;
y0.FromPrescan.Yaw_rate = 0;



if isempty(a)
    a = 1;
    y = y0;
    y.situationBus.wP.wayPointArray = veh_struct.initialWayPointsArray;
    y.situationBus.wP.currentWayPointIndex = veh_struct.initialCurrentWayPointIndex;
    y.situationBus.wP.finalWayPointIndex = veh_struct.initialFinalWayPointIndex;

else
    y = u;
end

== matlab function SingleVehicle_01/VehStateBusUnitDelayAndInit/MATLAB Function ==
  data: u input double; y output Bus: VehState
function y = DelayAndInitVehState(u)
persistent a
y0 = struct;
y0.x = 1;
y0.y = 2;
y0.z = 0;
y0.theta = 0;
y0.phi = 0;
y0.psi = 0;
y0.u = 0;
y0.v = 0;
y0.w = 0;
y0.dtheta = 0;
y0.dphi = 0;
y0.dpsi = 0;

% y0.PWAVehState = struct;
% y0.PWAVehState.Y_PWA = 0;
% y0.PWAVehState.vy_PWA = 0;
% y0.PWAVehState.yaw_angle_PWA = 0;
% y0.PWAVehState.yaw_rate_PWA = 0;

%y0 = VehState_MATLABStruct;
if isempty(a)
    a = 1;
    y = y0;
else
    y = u;
end

== matlab function SingleVehicle_01/Controller/SituationalAwareness/situationAwareness ==
  data: prevSituation input Bus: situationBus; newSituation output Bus: situationBus; prescanSimData input Bus: PrescanSimData; idealSensors input Bus: VehState; veh_struct parameter double
function newSituation = calcSituationAwareness(prevSituation,prescanSimData,idealSensors, veh_struct)

newSituation = prevSituation;


newSituation.selfAwarenessBus.x = idealSensors.x;
newSituation.selfAwarenessBus.y = idealSensors.y;
newSituation.selfAwarenessBus.z = idealSensors.z;
newSituation.selfAwarenessBus.theta = idealSensors.theta;
newSituation.selfAwarenessBus.phi = idealSensors.phi;
newSituation.selfAwarenessBus.psi = idealSensors.psi;
newSituation.selfAwarenessBus.u = idealSensors.u;
newSituation.selfAwarenessBus.v = idealSensors.v;
newSituation.selfAwarenessBus.w = idealSensors.w;
newSituation.selfAwarenessBus.dtheta = idealSensors.dtheta;
newSituation.selfAwarenessBus.dphi = idealSensors.dphi;
newSituation.selfAwarenessBus.dpsi = idealSensors.dpsi;

end

== matlab function SingleVehicle_01/Controller/FeaturedFunctions/wpFollower ==
  data: prevWpAction input Bus: wpFollower; prevSituation input Bus: situationBus; wpAction output Bus: wpFollower; veh_struct parameter double; newSituation output Bus: situationBus
function [wpAction, newSituation] = wpFollower(prevWpAction, prevSituation, veh_struct)

currentIndex = prevSituation.wP.currentWayPointIndex;
if currentIndex < 1
    currentIndex = uint16(1);
end
finalIndex = prevSituation.wP.finalWayPointIndex;

xd = prevSituation.wP.wayPointArray(currentIndex).x;
yd = prevSituation.wP.wayPointArray(currentIndex).y;
xa = prevSituation.selfAwarenessBus.x;
ya = prevSituation.selfAwarenessBus.y;
howClose = norm([xd-xa, yd-ya]);

if howClose < veh_struct.wpControl.wayPointThreshold
    if (currentIndex == finalIndex)
        currentIndex = uint16(1);
    else
        currentIndex = uint16(currentIndex + 1);
    end
end

newSituation = prevSituation;
newSituation.wP.currentWayPointIndex = uint16(currentIndex);
newSituation.wP.currentWayPoint.x = newSituation.wP.wayPointArray(currentIndex).x;
newSituation.wP.currentWayPoint.y = newSituation.wP.wayPointArray(currentIndex).y;
newSituation.wP.currentWayPoint.z = newSituation.wP.wayPointArray(currentIndex).z;
newSituation.wP.currentWayPoint.treach = newSituation.wP.wayPointArray(currentIndex).treach;

v_des_raw = min(veh_struct.wpControl.v_des_max, howClose / veh_struct.wpControl.howClose_saturate * veh_struct.wpControl.v_des_max);
psi_des_raw = atan2((yd-ya),(xd-xa));

% if psi_des_raw < 0
%     
%     dbg = 1;
%     
% end
    

v_des_old = prevWpAction.v_des;
psi_des_old = prevWpAction.psi_des;

a_des = veh_struct.wpControl.v_des_filter.lambda * (v_des_raw - v_des_old);
v_des = v_des_old + veh_struct.CONTROL_OS_SAMPLETIME * a_des;

dpsi_des = veh_struct.wpControl.psi_des_filter.lambda * (psi_des_raw - psi_des_old);
psi_des = psi_des_old + veh_struct.CONTROL_OS_SAMPLETIME * dpsi_des;
% psi_des = mod(psi_des, 2 * pi);


wpAction.v_des = v_des;
wpAction.a_des = a_des;
wpAction.psi_des = psi_des;
wpAction.dpsi_des = dpsi_des;

end

== matlab function SingleVehicle_01/Controller/StrategicArbitration/Arbitration ==
  data: FunctionFeatures input Bus: FunctionFeatures; ArbitratedReq output Bus: ArbitratedActuationReq
function ArbitratedReq = Arbitrate(FunctionFeatures)

ArbitratedReq.RHSCCmdBus.RHSC_steering_cmd = FunctionFeatures.RHSCCmdBus.RHSC_steering_cmd;
ArbitratedReq.v_des = FunctionFeatures.wpFollower.v_des;
ArbitratedReq.a_des = FunctionFeatures.wpFollower.a_des;
ArbitratedReq.psi_des = FunctionFeatures.wpFollower.psi_des;
ArbitratedReq.dpsi_des = FunctionFeatures.wpFollower.dpsi_des;



end

== matlab function SingleVehicle_01/Controller/Actuation/DynamicControls ==
  data: ActReq input Bus: ArbitratedActuationReq; Ctl input Bus: ControllerMainBus; ActCmds output Bus: ActuationCmdBus; ActCmdsPrev input Bus: ActuationCmdBus
function ActCmds  = fcn(ActReq, Ctl, ActCmdsPrev)

v_des = ActReq.v_des;
a_des = ActReq.a_des;
psi_des = ActReq.psi_des;
dpsi_des = ActReq.dpsi_des;

% ActCmds = ActCmdsPrev;
% ActCmds.accel_cmd = 0;
% ActCmds.decel_cmd = 0;
% ActCmds.steering_cmd = 0.1;

ActCmds = ActCmdsPrev;

if a_des >= 0
    ActCmds.accel_cmd = ActReq.a_des;
    ActCmds.decel_cmd = 0;
else
    ActCmds.accel_cmd = 0;
    ActCmds.decel_cmd = ActReq.a_des;
end

psi_des = unwrap(psi_des);
Ctl.IdealSensors.psi = unwrap(Ctl.IdealSensors.psi);

% ActCmds.steering_cmd = 3.5*(psi_des - Ctl.IdealSensors.psi);
ActCmds.steering_cmd = Ctl.FunctionFeatures.RHSCCmdBus.RHSC_steering_cmd;

== matlab function SingleVehicle_01/Controller/FeaturedFunctions/RHSC1 ==
  data: prevSituation input Bus: situationBus; preRHSCAction input Bus: RHSCCmdBus; RHSC_out output double; veh_struct parameter double
function RHSC_out = RHSC(prevSituation, preRHSCAction, veh_struct)

currentIndex = prevSituation.wP.currentWayPointIndex;
if currentIndex < 1
    currentIndex = uint16(1);
end
finalIndex = prevSituation.wP.finalWayPointIndex;

xd = prevSituation.wP.wayPointArray(currentIndex).x;
yd = prevSituation.wP.wayPointArray(currentIndex).y;
xa = prevSituation.selfAwarenessBus.x;
ya = prevSituation.selfAwarenessBus.y;
va = prevSituation.selfAwarenessBus.v;
psia = prevSituation.selfAwarenessBus.psi;
dpsia = prevSituation.selfAwarenessBus.dpsi;
oldu = preRHSCAction.RHSC_steering_cmd;

rou = veh_struct.RHSC.rou;

% optimization problem parameters
N = veh_struct.RHSC.N;%prediction horizon
T_s = veh_struct.RHSC.T_s;%sampling time
nx = veh_struct.RHSC.nx;% number of state varibles
nu = veh_struct.RHSC.nu;% number of inputs



yalmip('clear');
% optimization varibles define
uvar = sdpvar(repmat(nu,1,N+1),repmat(1,1,N+1));
xvar = sdpvar(repmat(nx,1,N+1),repmat(1,1,N+1));

alfa_f = sdpvar(repmat(1,1,N),repmat(1,1,N));
alfa_r = sdpvar(repmat(1,1,N),repmat(1,1,N));

Y_tgt = sdpvar(N+1,1);
% yaw_angle_tgt = sdpvar(N+1,1);
pastu = sdpvar(1);

s = sdpvar(repmat(1,1,N),repmat(1,1,N));

% system dynamics parameters
lf = veh_struct.lf_pwa;
lr = veh_struct.lr_pwa;
m = veh_struct.mass_pwa;
Iz = veh_struct.Iz_pwa;
C_f1 = veh_struct.Cf1_pwa;
C_r1 = veh_struct.Cr1_pwa;
C_f2 = veh_struct.Cf2_pwa;
C_r2 = veh_struct.Cr2_pwa;
C_f3 = veh_struct.Cf3_pwa;
C_r3 = veh_struct.Cr3_pwa;
bf1 = veh_struct.bf1_pwa;
br1 = veh_struct.br1_pwa;
bf2 = veh_struct.bf2_pwa;
br2 = veh_struct.br2_pwa;
bf3 = veh_struct.bf3_pwa;
br3 = veh_struct.br3_pwa;
f_thre = veh_struct.f_thre_pwa;
r_thre = veh_struct.r_thre_pwa;
vx = veh_struct.vx_pwa;

A11 = [1,T_s,T_s*vx,0;
    0,(C_f1+C_r1)/m/vx*T_s+1,0,((C_f1*lf-C_r1*lr)/m/vx-vx)*T_s;
    0,0,1,T_s;
    0,(C_f1*lf-C_r1*lr)/Iz/vx*T_s,0,(C_f1*lf^2+C_r1*lr^2)/Iz/vx*T_s+1];

A12 = [1,T_s,T_s*vx,0;
    0,(C_f1+C_r2)/m/vx*T_s+1,0,((C_f1*lf-C_r2*lr)/m/vx-vx)*T_s;
    0,0,1,T_s;
    0,(C_f1*lf-C_r2*lr)/Iz/vx*T_s,0,(C_f1*lf^2+C_r2*lr^2)/Iz/vx*T_s+1];

A13 = [1,T_s,T_s*vx,0;
    0,(C_f1+C_r3)/m/vx*T_s+1,0,((C_f1*lf-C_r3*lr)/m/vx-vx)*T_s;
    0,0,1,T_s;
    0,(C_f1*lf-C_r3*lr)/Iz/vx*T_s,0,(C_f1*lf^2+C_r3*lr^2)/Iz/vx*T_s+1];

A21 = [1,T_s,T_s*vx,0;
    0,(C_f2+C_r1)/m/vx*T_s+1,0,((C_f2*lf-C_r1*lr)/m/vx-vx)*T_s;
    0,0,1,T_s;
    0,(C_f2*lf-C_r1*lr)/Iz/vx*T_s,0,(C_f2*lf^2+C_r1*lr^2)/Iz/vx*T_s+1];

A22 = [1,T_s,T_s*vx,0;
    0,(C_f2+C_r2)/m/vx*T_s+1,0,((C_f2*lf-C_r2*lr)/m/vx-vx)*T_s;
    0,0,1,T_s;
    0,(C_f2*lf-C_r2*lr)/Iz/vx*T_s,0,(C_f2*lf^2+C_r2*lr^2)/Iz/vx*T_s+1];

A23 = [1,T_s,T_s*vx,0;
    0,(C_f2+C_r3)/m/vx*T_s+1,0,((C_f2*lf-C_r3*lr)/m/vx-vx)*T_s;
    0,0,1,T_s;
    0,(C_f2*lf-C_r3*lr)/Iz/vx*T_s,0,(C_f2*lf^2+C_r3*lr^2)/Iz/vx*T_s+1];

A31 = [1,T_s,T_s*vx,0;
    0,(C_f3+C_r1)/m/vx*T_s+1,0,((C_f3*lf-C_r1*lr)/m/vx-vx)*T_s;
    0,0,1,T_s;
    0,(C_f3*lf-C_r1*lr)/Iz/vx*T_s,0,(C_f3*lf^2+C_r1*lr^2)/Iz/vx*T_s+1];

A32 = [1,T_s,T_s*vx,0;
    0,(C_f3+C_r2)/m/vx*T_s+1,0,((C_f3*lf-C_r2*lr)/m/vx-vx)*T_s;
    0,0,1,T_s;
    0,(C_f3*lf-C_r2*lr)/Iz/vx*T_s,0,(C_f3*lf^2+C_r2*lr^2)/Iz/vx*T_s+1];

A33 = [1,T_s,T_s*vx,0;
    0,(C_f3+C_r3)/m/vx*T_s+1,0,((C_f3*lf-C_r3*lr)/m/vx-vx)*T_s;
    0,0,1,T_s;
    0,(C_f3*lf-C_r3*lr)/Iz/vx*T_s,0,(C_f3*lf^2+C_r3*lr^2)/Iz/vx*T_s+1];

B1 = [0;
    -C_f1/m*T_s;
    0;
    -lf*C_f1/Iz*T_s];

B2 = [0;
    -C_f2/m*T_s;
    0;
    -lf*C_f2/Iz*T_s];

B3 = [0;
    -C_f3/m*T_s;
    0;
    -lf*C_f3/Iz*T_s];

f11 = [0;
    T_s*(bf1+br1)/m;
    0;
    T_s*(lf*bf1-lr*br1)/Iz];

f12 = [0;
    T_s*(bf1+br2)/m;
    0;
    T_s*(lf*bf1-lr*br2)/Iz];

f13 = [0;
    T_s*(bf1+br3)/m;
    0;
    T_s*(lf*bf1-lr*br3)/Iz];

f21 = [0;
    T_s*(bf2+br1)/m;
    0;
    T_s*(lf*bf2-lr*br1)/Iz];

f22 = [0;
    T_s*(bf2+br2)/m;
    0;
    T_s*(lf*bf2-lr*br2)/Iz];

f23 = [0;
    T_s*(bf2+br3)/m;
    0;
    T_s*(lf*bf2-lr*br3)/Iz];

f31 = [0;
    T_s*(bf3+br1)/m;
    0;
    T_s*(lf*bf3-lr*br1)/Iz];

f32 = [0;
    T_s*(bf3+br2)/m;
    0;
    T_s*(lf*bf3-lr*br2)/Iz];

f33 = [0;
    T_s*(bf3+br3)/m;
    0;
    T_s*(lf*bf3-lr*br3)/Iz];

% problem formulation
constraints=[];
objective=0;

for k=1:N    
    
    alfa_f{k} = (xvar{k}(2)+lf*xvar{k}(4))/vx-uvar{k};
    
    alfa_r{k} = (xvar{k}(2)-lr*xvar{k}(4))/vx;
    
    s{k} = (xvar{k+1}(1)-Y_tgt(k+1))- rou*(xvar{k}(1)-Y_tgt(k));
    
    objective = objective + (s{k})^2;
    
    constraints = [constraints,-0.15 <= uvar{k} <= 0.15];
    
    constraints = [constraints,-0.05*0.1 <= uvar{k+1} -uvar{k} <=0.05*0.1];   
    
    constraints = [constraints,xvar{k+1} == A11*xvar{k} + B11*uvar{k} + f11]
    
    
end

    parameters_in = {xvar{1},Y_tgt,pastu};
    
    solutions_out = [uvar{1}];
    
    controller = optimizer(constraints,objective,parameters_in,[],solutions_out);    
    
    RHSC_out = controller{{[ya;va;psia;dpsia],yd*ones(N+1,1),oldu}};

end

== matlab function SingleVehicle_01/Controller/Actuation/ActuatorDrivers ==
  data: ActCmds input Bus: ActuationCmdBus; accel_cmd output double; decel_cmd output double; steering_cmd output double
function [accel_cmd, decel_cmd, steering_cmd]  = fcn(ActCmds)

accel_cmd = ActCmds.accel_cmd;
decel_cmd = ActCmds.decel_cmd;
steering_cmd = ActCmds.steering_cmd;

end

== matlab function SingleVehicle_01/VehicleDynamics/PWAVehicleDynamicsModel ==
  data: delta input double; dY output double; v input double; dv output double; psi input double; dpsi input double; veh_struct parameter double; ddpsi output double; mode output double
function [dY, dv, ddpsi, mode] = fcn(delta, v, psi, dpsi, veh_struct)
% persistent K_f K_r b_f b_r alfa_f alfa_r
lf = veh_struct.lf_pwa;
lr = veh_struct.lr_pwa;
m = veh_struct.mass_pwa;
Iz = veh_struct.Iz_pwa;
C_f1 = veh_struct.Cf1_pwa;
C_r1 = veh_struct.Cr1_pwa;
C_f2 = veh_struct.Cf2_pwa;
C_r2 = veh_struct.Cr2_pwa;
C_f3 = veh_struct.Cf3_pwa;
C_r3 = veh_struct.Cr3_pwa;
bf1 = veh_struct.bf1_pwa;
br1 = veh_struct.br1_pwa;
bf2 = veh_struct.bf2_pwa;
br2 = veh_struct.br2_pwa;
bf3 = veh_struct.bf3_pwa;
br3 = veh_struct.br3_pwa;
f_thre = veh_struct.f_thre_pwa;
r_thre = veh_struct.r_thre_pwa;
vx = veh_struct.vx_pwa;

K_f = 0;
K_r = 0;
b_f = 0;
b_r = 0;
mode = 0;

alfa_f = (v + dpsi*lf)/vx - delta;
alfa_r = (v - dpsi*lr)/vx;

% K_f = C_f1;
% K_r = C_r1;
% b_f = bf1;
% b_r = br1;
if ((-f_thre <= alfa_f) && (alfa_f <= f_thre)) && ((-r_thre<= alfa_r) && (alfa_r <=r_thre))
    K_f = C_f1;
    K_r = C_r1;
    b_f = bf1;
    b_r = br1;
    mode = 1;
else if ((-f_thre <= alfa_f) && (alfa_f <= f_thre)) && (alfa_r <= -r_thre)
        K_f = C_f1;
        K_r = C_r2;
        b_f = bf1;
        b_r = br2;
        mode = 2;
    else if ((-f_thre <= alfa_f) && (alfa_f <= f_thre)) && (alfa_r >= r_thre)
            K_f = C_f1;
            K_r = C_r3;
            b_f = bf1;
            b_r = br3;
            mode = 3;
        else if ((alfa_f <= -f_thre) && ((-r_thre<= alfa_r) && (alfa_r <=r_thre)))
                K_f = C_f2;
                K_r = C_r1;
                b_f = bf2;
                b_r = br1;
                mode = 4;
            else if (alfa_f <= -f_thre) && (alfa_r <= -r_thre)
                    K_f = C_f2;
                    K_r = C_r2;
                    b_f = bf2;
                    b_r = br2;
                    mode = 5;
                else if (alfa_f <= -f_thre) && (alfa_r >= r_thre)
                        K_f = C_f2;
                        K_r = C_r3;
                        b_f = bf2;
                        b_r = br3;
                        mode = 6;
                    else if (alfa_f >= f_thre) && ((-r_thre<= alfa_r) && (alfa_r <=r_thre))
                            K_f = C_f3;
                            K_r = C_r1;
                            b_f = bf3;
                            b_r = br1;
                            mode = 7;
                        else if (alfa_f >= f_thre) && (alfa_r <= -r_thre)
                                K_f = C_f3;
                                K_r = C_r2;
                                b_f = bf3;
                                b_r = br2;
                                mode = 8;
                            else if (alfa_f >= f_thre) && (alfa_r >= r_thre)
                                    K_f = C_f3;
                                    K_r = C_r3;
                                    b_f = bf3;
                                    b_r = br3;
                                    mode = 9;
                                end
                            end
                        end
                    end
                end
            end
        end
    end
end


dY = vx*psi + v;
dv = (K_f + K_r)/m/vx*v + ((K_f*lf - K_r*lr)/m/vx - vx)*dpsi - K_f/m*delta + (b_f + b_r)/m;
ddpsi = (K_f*lf - K_r*lr)/Iz/vx*v + (K_f*lf^2 + K_r*lr^2)/Iz/vx*dpsi - K_f*lf/Iz*delta + (b_f*lf - b_r*lr)/Iz;
